simulink model "bo1808_svpwm_sfunc_sim"  (R2024b)
settings: Solver=ode23tb  StartTime=0.0  StopTime=t_stop_svpwm  MaxStep=Ts_sim_svpwm  RelTol=1e-3
model workspace (MAT data in the model file):
  Ts_pwm_svpwm = 5e-05
  Ts_sim_svpwm = 1e-06
  Uref_svpwm = 4.83590678003
  Vdc = 11.4
  Vref_max_svpwm = 6.58179306876
  f_ref_svpwm = 519.333333333
  fft_cycles_svpwm = 20
  fs_pwm = 20000
  id_ref_svpwm = 0
  iq_ref_svpwm = 0.1875
  m_svpwm = 0.734740021375
  omega_ref_svpwm = 3263.06756953
  t_stop_svpwm = 0.0385109114249
  ud_ref_svpwm = -0.226375312636
  uq_ref_svpwm = 4.8306054075
libraries: simulink x1
settings Model: Creator=26683  LastModifiedBy=26683

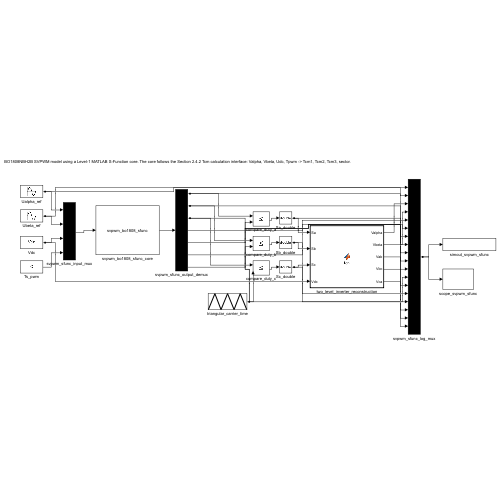
[thumbnail: Simulink's stored preview of the top-level diagram]
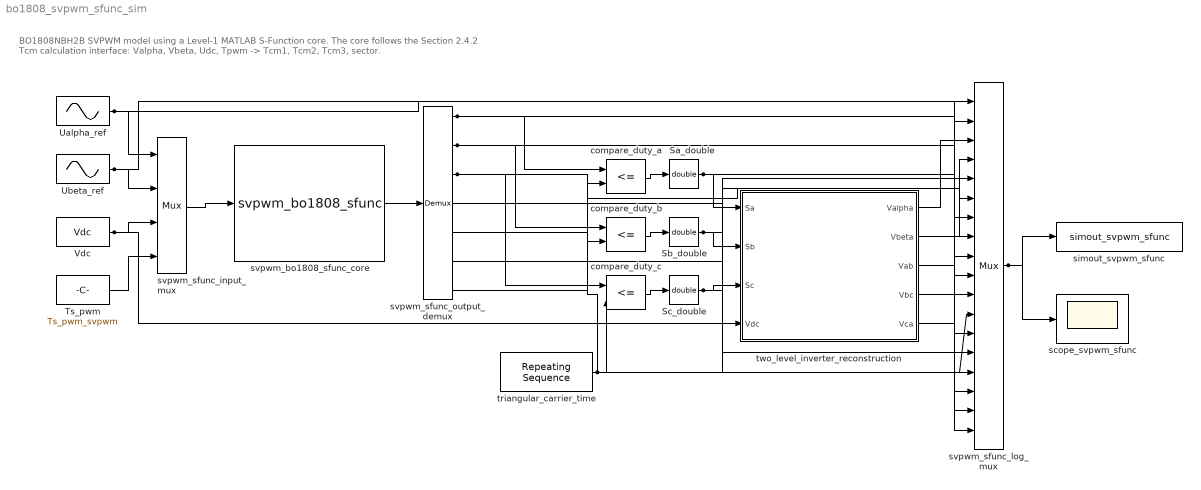
== system bo1808_svpwm_sfunc_sim ==
  note: BO1808NBH2B SVPWM model using a Level-1 MATLAB S-Function core. The core follows the Section 2.4.2 Tcm calculation interface: Valpha, Vbeta, Udc, Tpwm -> Tcm1, Tcm2, Tcm3, sector.
  Sa_double : DataTypeConversion  OutDataTypeStr=double  SaturateOnIntegerOverflow=off  RndMeth=Floor
  Sb_double : DataTypeConversion  OutDataTypeStr=double  SaturateOnIntegerOverflow=off  RndMeth=Floor
  Sc_double : DataTypeConversion  OutDataTypeStr=double  SaturateOnIntegerOverflow=off  RndMeth=Floor
  Ts_pwm : Constant  Value=Ts_pwm_svpwm
  Ualpha_ref : Sin  Amplitude=Uref_svpwm  Frequency=2*pi*f_ref_svpwm  Phase=pi/2  SampleTime=0
  Ubeta_ref : Sin  Amplitude=Uref_svpwm  Frequency=2*pi*f_ref_svpwm  SampleTime=0
  Vdc : Constant  Value=Vdc
  compare_duty_a : RelationalOperator  Operator=<=  OutDataTypeStr=boolean  RndMeth=Simplest  InputSameDT=off
  compare_duty_b : RelationalOperator  Operator=<=  OutDataTypeStr=boolean  RndMeth=Simplest  InputSameDT=off
  compare_duty_c : RelationalOperator  Operator=<=  OutDataTypeStr=boolean  RndMeth=Simplest  InputSameDT=off
  scope_svpwm_sfunc : Scope
  simout_svpwm_sfunc : ToWorkspace  VariableName=simout_svpwm_sfunc  SaveFormat=Structure With Time  SampleTime=-1
  svpwm_bo1808_sfunc_core : S-Function  FunctionName=svpwm_bo1808_sfunc  SFunctionDeploymentMode=off  EnableBusSupport=off
  svpwm_sfunc_input_mux : Mux
  svpwm_sfunc_log_mux : Mux  Inputs=18
  svpwm_sfunc_output_demux : Demux  Outputs=7
  triangular_carrier_time : simulink/Sources/Repeating Sequence  rep_seq_t=[0 Ts_pwm_svpwm/2 Ts_pwm_svpwm]  rep_seq_y=[0 Ts_pwm_svpwm/2 0]
  two_level_inverter_reconstruction : MATLAB Function  TreatAsAtomicUnit=on
  wires:
  Ualpha_ref/1 -> svpwm_sfunc_input_mux/1, svpwm_sfunc_log_mux/1
  Ubeta_ref/1 -> svpwm_sfunc_input_mux/2, svpwm_sfunc_log_mux/2
  Vdc/1 -> svpwm_sfunc_input_mux/3, two_level_inverter_reconstruction/4(Vdc)
  Ts_pwm/1 -> svpwm_sfunc_input_mux/4
  svpwm_sfunc_input_mux/1 -> svpwm_bo1808_sfunc_core/1
  svpwm_bo1808_sfunc_core/1 -> svpwm_sfunc_output_demux/1
  svpwm_sfunc_output_demux/1 -> compare_duty_a/1, svpwm_sfunc_log_mux/9
  svpwm_sfunc_output_demux/2 -> compare_duty_b/1, svpwm_sfunc_log_mux/10
  svpwm_sfunc_output_demux/3 -> compare_duty_c/1, svpwm_sfunc_log_mux/11
  triangular_carrier_time/1 -> compare_duty_a/2, compare_duty_b/2, compare_duty_c/2, svpwm_sfunc_log_mux/12
  compare_duty_a/1 -> Sa_double/1
  compare_duty_b/1 -> Sb_double/1
  compare_duty_c/1 -> Sc_double/1
  Sa_double/1 -> two_level_inverter_reconstruction/1(Sa), svpwm_sfunc_log_mux/13
  Sb_double/1 -> two_level_inverter_reconstruction/2(Sb), svpwm_sfunc_log_mux/14
  Sc_double/1 -> two_level_inverter_reconstruction/3(Sc), svpwm_sfunc_log_mux/15
  two_level_inverter_reconstruction/1(Valpha) -> svpwm_sfunc_log_mux/3
  two_level_inverter_reconstruction/2(Vbeta) -> svpwm_sfunc_log_mux/4
  svpwm_sfunc_output_demux/4 -> svpwm_sfunc_log_mux/5
  svpwm_sfunc_output_demux/5 -> svpwm_sfunc_log_mux/6
  svpwm_sfunc_output_demux/6 -> svpwm_sfunc_log_mux/7
  svpwm_sfunc_output_demux/7 -> svpwm_sfunc_log_mux/8
  two_level_inverter_reconstruction/3(Vab) -> svpwm_sfunc_log_mux/16
  two_level_inverter_reconstruction/4(Vbc) -> svpwm_sfunc_log_mux/17
  two_level_inverter_reconstruction/5(Vca) -> svpwm_sfunc_log_mux/18
  svpwm_sfunc_log_mux/1 -> simout_svpwm_sfunc/1, scope_svpwm_sfunc/1

== matlab function bo1808_svpwm_sfunc_sim/two_level_inverter_reconstruction ==
  data: Sa input; Valpha output; Sb input; Sc input; Vdc input; Vbeta output; Vab output; Vbc output; Vca output
function [Valpha,Vbeta,Vab,Vbc,Vca] = fcn(Sa,Sb,Sc,Vdc)
%#codegen
sa = double(Sa);
sb = double(Sb);
sc = double(Sc);
Va0 = (sa - 0.5)*Vdc;
Vb0 = (sb - 0.5)*Vdc;
Vc0 = (sc - 0.5)*Vdc;
Vab = Va0 - Vb0;
Vbc = Vb0 - Vc0;
Vca = Vc0 - Va0;
Valpha = (2/3)*(Va0 - 0.5*Vb0 - 0.5*Vc0);
Vbeta = (2/3)*(sqrt(3)/2)*(Vb0 - Vc0);
end
